simulink model "Symulacja_URA_na_podstawie_aktualnego_TP"  (R2022b)
settings: Solver=VariableStepAuto  StartTime=0.0  StopTime=100  RelTol=1e-3
settings Model: Creator=hpiet  LastModifiedBy=hpiet
settings DebuggingCC: UnderSpecifiedDimensionMsg=warning

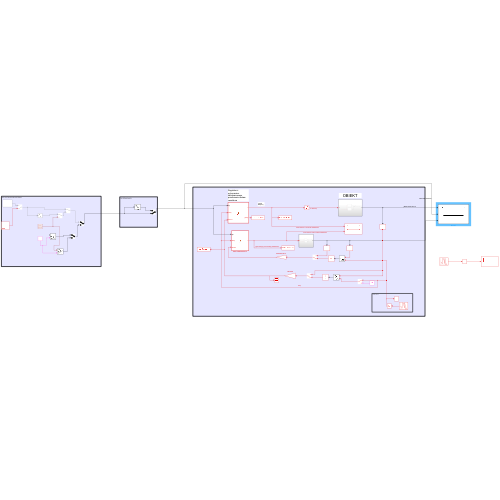
[thumbnail: Simulink's stored preview of the top-level diagram]
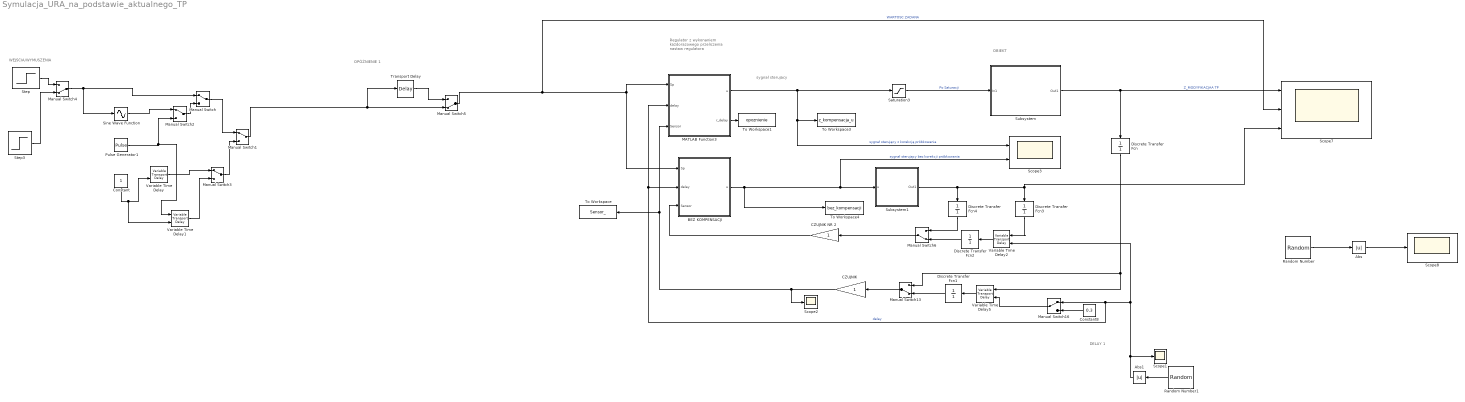
== system Symulacja_URA_na_podstawie_aktualnego_TP ==
  note: OBIEKT
  note: DELAY 1
  note: sygnał sterujacy
  note: Regulator z wykonaniem każdorazowego przeliczenia nastaw regulatora
  note: WEJŚĆIA/WYMUSZENIA
  note: OPÓŹNIENIE 1
  Abs : Abs  SaturateOnIntegerOverflow=off
  Abs1 : Abs  SaturateOnIntegerOverflow=off
  BEZ KOMPENSACJI : MATLAB Function  TreatAsAtomicUnit=on
  CZUJNIK : Gain
  CZUJNIK NR 2 : Gain
  Constant : Constant
  Constant8 : Constant  Value=0.3
  Discrete Transfer Fcn{,1..4} (5 alike) : DiscreteTransferFcn  Denominator=[1]
  MATLAB Function3 : MATLAB Function  TreatAsAtomicUnit=on
  Manual Switch{,1..3,16} (5 alike) : ManualSwitch
  Manual Switch{4..6,13} (4 alike) : ManualSwitch  CurrentSetting=0
  Pulse Generator1 : DiscretePulseGenerator  PulseType=Time based  Period=10  PulseWidth=90
  Random Number : RandomNumber  Variance=0.02  SampleTime=0.1
  Random Number1 : RandomNumber  Mean=0.2  Variance=0.0001  SampleTime=0.1
  Saturation3 : Saturate  UpperLimit=1200  LowerLimit=0
  Scope1 : Scope
  Scope2 : Scope
  Scope3 : Scope  NumInputPorts=2
  Scope7 : Scope  NumInputPorts=3
  Scope8 : Scope
  Sine Wave Function : Sin  TimeSource=Use external signal  SampleTime=0
  Step : Step  Time=0  After=1100  SampleTime=0
  Step3 : Step  Time=0  After=25  SampleTime=0.1
  Subsystem : Subsystem
  Subsystem1 : Subsystem
  To Workspace : ToWorkspace  VariableName=Sensor_  SaveFormat=Structure With Time  SampleTime=-1
  To Workspace1 : ToWorkspace  VariableName=opoznienie  SaveFormat=Timeseries  SampleTime=-1
  To Workspace3 : ToWorkspace  VariableName=z_kompensacja_u  SaveFormat=Timeseries  SampleTime=-1
  To Workspace4 : ToWorkspace  VariableName=bez_kompensacji  SaveFormat=Timeseries  SampleTime=-1
  Transport Delay : TransportDelay  DelayTime=0.012
  Variable Time Delay{,1..2,5} (4 alike) : VariableTransportDelay  MaximumDelay=10
  wires:
  Constant8/1 -> Manual Switch16/2
  Random Number1/1 -> Abs1/1
  Manual Switch16/1 -> Variable Time Delay5/2
  Random Number/1 -> Abs/1
  Saturation3/1 -> Subsystem/1(In1)  "Po Saturacji"
  Abs/1 -> Scope8/1
  CZUJNIK/1 -> MATLAB Function3/3(Sensor), To Workspace/1, Scope2/1
  MATLAB Function3/1(u) -> Scope3/1, To Workspace3/1, Saturation3/1  "sygnał sterujący z korekcją próbkowania"
  Manual Switch13/1 -> CZUJNIK/1
  Subsystem/1(Out1) -> Discrete Transfer Fcn/1, Scope7/1  "Z_MODYFIKACJAA TP"
  Variable Time Delay5/1 -> Discrete Transfer Fcn1/1
  Abs1/1 -> Scope1/1, MATLAB Function3/2(delay), BEZ KOMPENSACJI/2(delay), Manual Switch16/1, Variable Time Delay2/2  "delay"
  Constant/1 -> Variable Time Delay1/2, Variable Time Delay/2
  Variable Time Delay1/1 -> Manual Switch3/2
  Manual Switch3/1 -> Manual Switch1/2
  Step3/1 -> Manual Switch4/2
  Step/1 -> Manual Switch4/1
  Pulse Generator1/1 -> Variable Time Delay1/1, Manual Switch2/2
  Variable Time Delay/1 -> Manual Switch3/1
  Sine Wave Function/1 -> Manual Switch2/1
  Manual Switch/1 -> Manual Switch1/1
  Manual Switch1/1 -> Manual Switch5/2, Transport Delay/1
  Manual Switch2/1 -> Manual Switch/2
  Manual Switch4/1 -> Sine Wave Function/1, Manual Switch/1
  Transport Delay/1 -> Manual Switch5/1
  Manual Switch5/1 -> Scope7/2, MATLAB Function3/1(Sp), BEZ KOMPENSACJI/1(Sp)  "WARTOSC ZADANA"
  Discrete Transfer Fcn/1 -> Variable Time Delay5/1, Manual Switch13/1
  Discrete Transfer Fcn1/1 -> Manual Switch13/2
  MATLAB Function3/2(r_delay) -> To Workspace1/1
  BEZ KOMPENSACJI/1(u) -> Scope3/2, Subsystem1/1(u), To Workspace4/1  "sygnał sterujący bez korekcji próbkowania"
  Subsystem1/1(Out1) -> Scope7/3, Discrete Transfer Fcn3/1, Discrete Transfer Fcn4/1
  Variable Time Delay2/1 -> Discrete Transfer Fcn2/1
  Discrete Transfer Fcn2/1 -> Manual Switch6/2
  Manual Switch6/1 -> CZUJNIK NR 2/1
  CZUJNIK NR 2/1 -> BEZ KOMPENSACJI/3(Sensor)
  Discrete Transfer Fcn3/1 -> Variable Time Delay2/1
  Discrete Transfer Fcn4/1 -> Manual Switch6/1

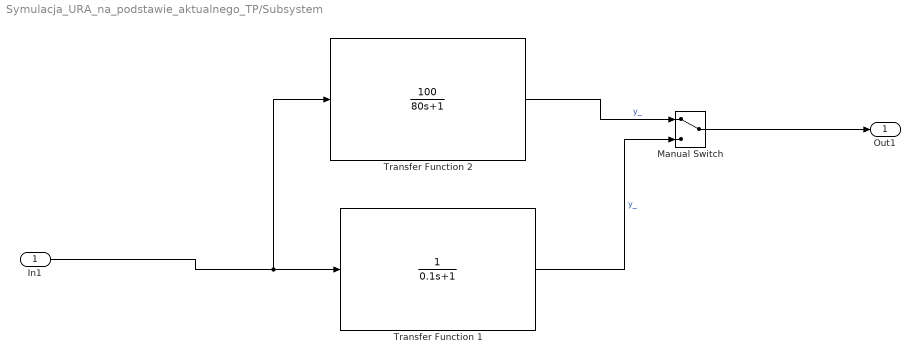
== system Symulacja_URA_na_podstawie_aktualnego_TP/Subsystem ==
  In1 : Inport
  Manual Switch : ManualSwitch
  Transfer Function 1 : TransferFcn  Denominator=[0.1 1]
  Transfer Function 2 : TransferFcn  Numerator=[100]  Denominator=[80 1]
  Out1 : Outport
  wires:
  In1/1 -> Transfer Function 2/1, Transfer Function 1/1
  Transfer Function 1/1 -> Manual Switch/2  "y_"
  Transfer Function 2/1 -> Manual Switch/1  "y_"
  Manual Switch/1 -> Out1/1

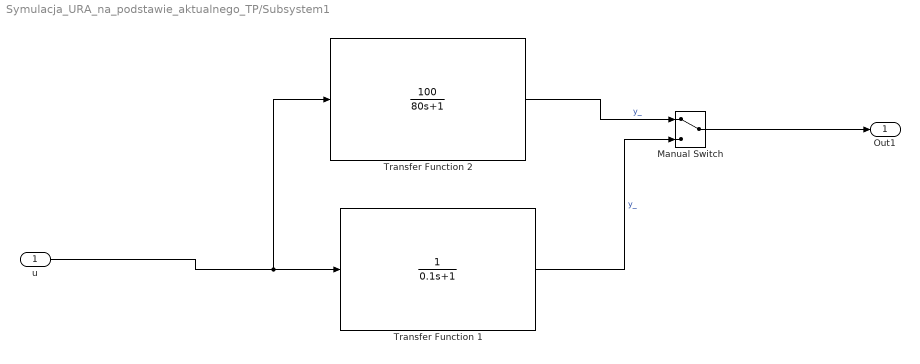
== system Symulacja_URA_na_podstawie_aktualnego_TP/Subsystem1 ==
  u : Inport
  Manual Switch : ManualSwitch
  Transfer Function 1 : TransferFcn  Denominator=[0.1 1]
  Transfer Function 2 : TransferFcn  Numerator=[100]  Denominator=[80 1]
  Out1 : Outport
  wires:
  u/1 -> Transfer Function 2/1, Transfer Function 1/1
  Transfer Function 1/1 -> Manual Switch/2  "y_"
  Transfer Function 2/1 -> Manual Switch/1  "y_"
  Manual Switch/1 -> Out1/1

== matlab function Symulacja_URA_na_podstawie_aktualnego_TP/BEZ KOMPENSACJI ==
  settings: updateMethod=DISCRETE
  data: Sp input; u output; delay input; Sensor input
function u= fcn(Sp,delay,Sensor) %wyjscie = funkcja(wejscia)
persistent init e2 e1 u2 u1 ku1 ku2 ke0 ke1 ke2 ;

if isempty(init) %wykonuje się tylko raz
Kp = 0.0975043176181261;
Ki =0.00404938736460088;
Kd = 0.148625801524361;
FCoef = 0.191342781331139;


Ts=0.1; %czas próbki
%TsReal=Ts+delay;


e2=0;
e1=0;
u2=0;
u1=0;

a0 = (1 + FCoef * Ts);
a1 = -(2 + FCoef * Ts);
a2 = 1;

b0=Kp*(1+FCoef * Ts) + Ki*Ts*(1+ FCoef*Ts) + Kd*FCoef;
b1= -(Kp*(2+FCoef*Ts) + Ki*Ts + 2*Kd*FCoef);
b2=Kp + Kd * FCoef;


%TEST
% a0 = (1 + FCoef * TsReal);
% a1 = -(2 + FCoef * TsReal);
% a2 = 1;
% 
% b0=Kp*(1+FCoef * TsReal) + Ki*TsReal*(1+ FCoef*TsReal) + Kd*FCoef;
% b1= -(Kp*(2+FCoef*TsReal) + Ki*TsReal + 2*Kd*FCoef);
% b2=Kp + Kd * FCoef;


%uproszczenie równania
ku1=a1/a0;
ku2=a2/a0;
ke0=b0/a0;
ke1=b1/a0;
ke2=b2/a0;

init=1;
end

e0 = Sp-Sensor;
u0 = -(ku1*u1) - (ku2 * u2) + (ke0*e0) + (ke1*e1) + (ke2*e2);

e2=e1;
e1=e0;
u2=u1;
u1=u0;

u=u0;



end

== matlab function Symulacja_URA_na_podstawie_aktualnego_TP/MATLAB Function3 ==
  settings: updateMethod=DISCRETE
  data: Sp input; u output; delay input; Sensor input; r_delay output
 function [u,r_delay]= fcn(Sp,delay,Sensor) %wyjscie = funkcja(wejscia)
persistent init e2 e1 u2 u1 ku1 ku2 ke0 ke1 ke2 actualTp i time_vec previousTp Kp Ki Kd FCoef;

if isempty(init) %wykonuje się tylko raz
Kp = 0.0975043176181261;
Ki =0.00404938736460088;
Kd = 0.148625801524361;
FCoef = 0.191342781331139;

% DO WYWALENIA
actualTp=0.1;

%DO SPRAWDZANIA
i=0.1;
time_vec=0;

e2=0;
e1=0;
u2=0;
u1=0;

init=1;
end

%MODYFIKACJA TP
actualTp=i+delay;
time_vec = [time_vec,actualTp];
previousTp=time_vec(end-1);

CorrectedTp = actualTp - previousTp

% disp('aktualna chwila czasowa')
% disp(actualTp)
% disp('Ostatnia chwila czasowa:')
% disp(previousTp)
disp('TIMESTAMP diff')
disp(CorrectedTp)


%TEST
a0 = (1 + FCoef * CorrectedTp);
a1 = -(2 + FCoef * CorrectedTp);
a2 = 1;

b0=Kp*(1+FCoef * CorrectedTp) + Ki*CorrectedTp*(1+ FCoef*CorrectedTp) + Kd*FCoef;
b1= -(Kp*(2+FCoef*CorrectedTp) + Ki*CorrectedTp + 2*Kd*FCoef);
b2=Kp + Kd * FCoef;


%uproszczenie równania
ku1=a1/a0;
ku2=a2/a0;
ke0=b0/a0;
ke1=b1/a0;
ke2=b2/a0;

e0 = Sp-Sensor;
%disp(Sensor)
u0 = -(ku1*u1) - (ku2 * u2) + (ke0*e0) + (ke1*e1) + (ke2*e2);

e2=e1;
e1=e0;
u2=u1;
u1=u0;

u=u0;
r_delay=delay;
i=i+0.1;

end
